simulink model "FOC_Ctrl_MBD"  (R2025b)
settings: Solver=FixedStepDiscrete  StartTime=0.0  StopTime=10.0  FixedStep=Ts  RelTol=1e-3
InitFcn:
  | mbd_s32k_consistency_checks(bdroot(gcs));
undefined symbols (not defined in the file): External, LQFP, One, Shot, TRGMUX_PDB_TRIG
libraries: mbd_s32k1xx_ec_toolbox x34, mbd_msd_ec_toolbox x1
settings Model: Creator=k  LastModifiedBy=k
settings SolverCC: AlgebraicLoopSolver=TrustRegion
settings DataIOCC: ExternalInput=off  InitialState=off  SaveOutput=off  SignalLogging=off  SaveTime=off
settings OptimizationCC: DefaultParameterBehavior=Inlined  StrengthReduction=on  PassReuseOutputArgsAs=Individual arguments  ZeroExternalMemoryAtStartup=off  ZeroInternalMemoryAtStartup=off  OptimizeBlockOrder=speed  OptimizationPriority=Speed  OptimizationCustomize=off  MultiThreadedLoops=on  AutoScheduleForLoops=on  EfficientTunableParamExpr=on
settings DebuggingCC: InheritedTsInSrcMsg=none  SingleTaskRateTransMsg=error  ParameterTunabilityLossMsg=error  UnconnectedInputMsg=error  UnconnectedOutputMsg=error  UnconnectedLineMsg=error  UnknownTsInhSupMsg=error
settings HardwareCC: ProdBitPerPointer=32.0  ProdBitPerSizeT=32.0  ProdBitPerPtrDiffT=32.0  ProdLargestAtomicInteger=Long  ProdLargestAtomicFloat=Double  ProdWordSize=32.0  ProdHWDeviceType=ARM Compatible->ARM Cortex
settings ModelReferenceCC: EnableRefExpFcnMdlSchedulingChecks=on  ModelReferenceNumInstancesAllowed=Single
settings SFSimCC: MATLABDynamicMemAlloc=off
settings RTWCC: SystemTargetFile=mbd_s32k.tlc  MakeCommand=mbd_s32k_make_rtw COPY_MDLREF_INCLUDES=0  TemplateMakefile=mbd_s32k.tmf  GenerateReport=on  GPUComputeCapability=3.5  DLArmComputeVersion=19.05  Description=Model Based Design Toolbox S32K1xx Code Generation Target
settings CodeAppCC: ForceParamTrailComments=on  IgnoreCustomStorageClasses=off  OperatorAnnotations=on  SimulinkDataObjDesc=on  SFDataObjDesc=on  InsertBlockDesc=on
settings STFCustomTargetCC: SystemTargetFile=mbd_s32k.tlc  TargetLangStandard=C99 (ISO)  MultiwordLength=256.0  ConcurrentExecutionCompliant=off  CombineOutputUpdateFcns=on  ERTCustomFileBanners=on  SubcomponentCodeInterfacePackaging=Nonreusable function  SupportContinuousTime=off  SupportNonInlinedSFcns=off  RemoveResetFunc=on  MATLABClassNameForMDSCustomization=Simulink.SoftwareTarget.ERTCustomization  GRTInterface=off
settings ERTTargetCC: ERTSrcFileBannerTemplate=mbd_ert_code_template.cgt  ERTHdrFileBannerTemplate=mbd_ert_code_template.cgt  ERTDataSrcFileTemplate=mbd_ert_code_template.cgt  ERTDataHdrFileTemplate=mbd_ert_code_template.cgt  ERTCustomFileTemplate=example_file_process.tlc  DynamicArrayContainerType=coder::array  TargetLangStandard=C99 (ISO)  ParMdlRefBuildCompliant=off  CompOptLevelCompliant=off  ConcurrentExecutionCompliant=off  SubcomponentCodeInterfacePackaging=Nonreusable function  ModelStepFunctionPrototypeControlCompliant=off  CPPClassGenCompliant=off  UseToolchainInfoCompliant=off

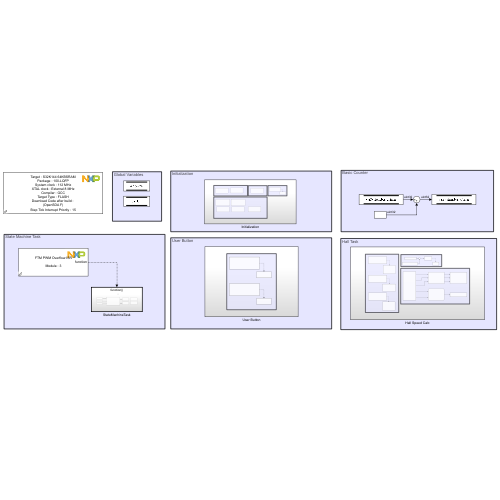
[thumbnail: Simulink's stored preview of the top-level diagram]
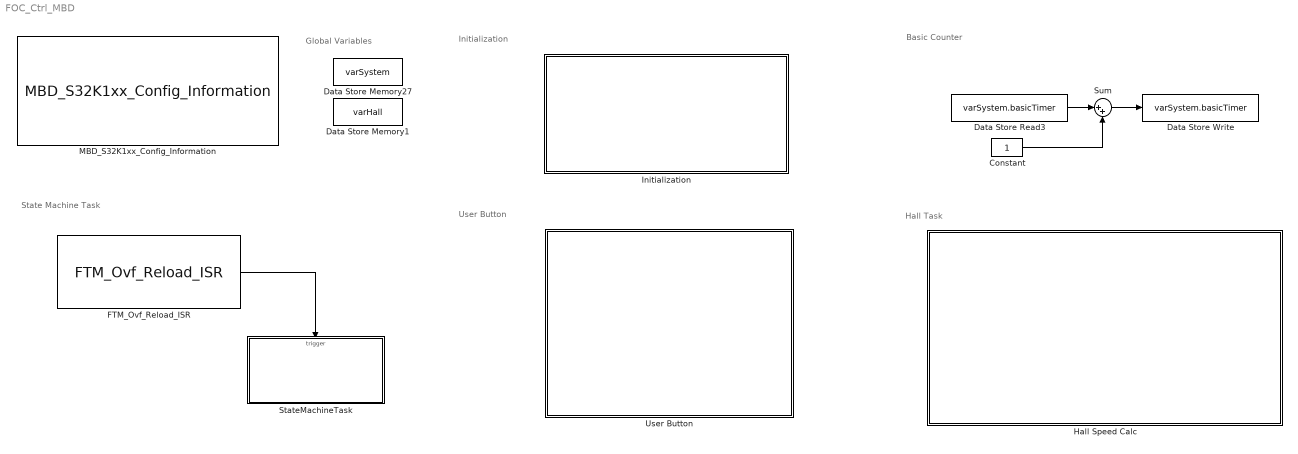
== system FOC_Ctrl_MBD ==
  note: Hall Task
  note: State Machine Task
  note: Global Variables
  note: User Button
  note: Initialization
  note: Basic Counter
  Constant : Constant  OutDataTypeStr=uint32
  Data Store Memory1 : DataStoreMemory  DataStoreName=varHall  ReadBeforeWriteMsg=warning  WriteAfterWriteMsg=warning  WriteAfterReadMsg=warning  ShowAdditionalParam=off  OutDataTypeStr=Bus: structHall
  Data Store Memory27 : DataStoreMemory  DataStoreName=varSystem  ReadBeforeWriteMsg=warning  WriteAfterWriteMsg=warning  WriteAfterReadMsg=warning  ShowAdditionalParam=off  OutDataTypeStr=Bus: structSystem
  Data Store Read3 : DataStoreRead  DataStoreName=varSystem  DataStoreElements=varSystem.basicTimer  IndexOptions=Index vector (dialog)  Indices=1  OutputSizes=1
  Data Store Write : DataStoreWrite  DataStoreName=varSystem  DataStoreElements=varSystem.basicTimer  IndexOptions=Index vector (dialog)  Indices=1  OutputSizes=1
  FTM_Ovf_Reload_ISR : mbd_s32k1xx_ec_toolbox/Motor Control Blocks/FTM Blocks/FTM_Ovf_Reload_ISR  Priority=10  ftmModule=3  mcuTargetUpdate=on
  Hall Speed Calc : Subsystem
  Initialization : Subsystem
  MBD_S32K1xx_Config_Information : mbd_s32k1xx_ec_toolbox/MBD_S32K1xx_Config_Information  mbdt_ver=0  disp_str=|  config_params=[]  mcu_target_name=S32K144  mcu_target_package=100-LQFP  mcu_target_sram_size=64KB  mcu_system_clock_freq=112  mcu_xtal_freq=External 8  mcu_steptick_timer=LPIT Channel 0  mcu_steptick_prio=15  ds_import_enable=on  target_compiler=GCC  target_memory=FLASH  gcc_target_compile_opts=-mthumb -mfloat-abi=hard -mfpu=fpv4-sp-d16 -O1 -g -gstrict-dwarf  gcc_target_assemble_opts=-mthumb -mfloat-abi=hard -mfpu=fpv4-sp-d16 -g  gcc_target_link_opts=-mthumb -mfloat-abi=hard -mfpu=fpv4-sp-d16  gcc_target_default_lcf=on  gcc_target_user_lcf=S32K144_64_flash.ld  ghs_target_compile_opts=-cpu=cortexm4f -thumb -fpu=vfpv4_d16 -fsingle -Ogeneral -Wundef -Wimplicit-int -Wshadow -Wtrigraphs --no_commons --gnu_asm -gnu99 -gdwarf-2 -G  ghs_target_assemble_opts=-cpu=cortexm4f -fpu=vfpv4_d16  ghs_target_link_opts=-cpu=cortexm4f -thumb -fpu=vfpv4_d16  ghs_target_default_lcf=on  ghs_target_user_lcf=S32K144_64_flash.ld  iar_target_compile_opts=--cpu=Cortex-M4F --thumb --fpu=VFPv4_sp -Ol -e --debug --dlib_config normal  iar_target_assemble_opts=--cpu Cortex-M4F --thumb --fpu VFPv4_sp  iar_target_link_opts=--no_exceptions --vfe --inline  iar_target_default_lcf=on  iar_target_user_lcf=S32K144_64_flash.icf  pil_download_enable=off  rbl_download_enable=on  rbl_start_delay=5000  rbl_download_interface=OpenSDA  rbl_restart_request=off  rbl_com_port=Custom  rbl_com_port_custom=COM1  pil_download_rate=57600  pil_download_rate_custom=115200  pil_opensda_drive=Custom  pil_opensda_drive_custom=F  jtag_interface=SEGGER JLink  jlink_default_path=off  jlink_user_path=C:\Program Files\SEGGER\JLink_V928  pil_uart_instance=1  pil_uart_rx=PTC6: [LPUART1_RX | Receive]  pil_uart_tx=PTC7: [LPUART1_TX | Transmit]  FTM_PWM_PcrCheckEnDis=on  FTM_Input_Edge_Inputs_PcrCheckEnDis=on  FTM_Dual_Edge_Inputs_PcrCheckEnDis=on  FTM_Quadrature_Inputs_PcrCheckEnDis=on  FTM_Hall_Sensor_Inputs_PcrCheckEnDis=on  LPTMR_PcrCheckEnDis=on  PIT_PcrCheckEnDis=on  RTC_PcrCheckEnDis=on  FlexCAN_PcrCheckEnDis=on  LIN_PcrCheckEnDis=on  FlexIO_PcrCheckEnDis=on  LPI2C_PcrCheckEnDis=on  LPSPI_PcrCheckEnDis=on  LPUART_PcrCheckEnDis=on  CMP_PcrCheckEnDis=on  GPIO_OutputPcrCheckEnDis=on  GPIO_InputPcrCheckEnDis=on  SBC_PcrCheckEnDis=on  BMS_PcrCheckEnDis=on  AMMCLIB_PcrCheckEnDis=on  FM_PcrCheckEnDis=on  Profile_PcrCheckEnDis=on  ConfigParams_PcrCheckEnDis=on  ModelRef_PcrCheckEnDis=on  PDB0_PcrCheckEnDis=on  CSEc_PcrCheckEnDis=on  eDMA_PcrCheckEnDis=on  FLASH_PcrCheckEnDis=on  ADC_PcrCheckEnDis=on  WDOG_PcrCheckEnDis=on
      | Target : S32K144-64KB_SRAM
      | Package : 100-pin
      | System clock : 80 MHz
      | XTAL clock : External 8 MHz
      | Compiler : IAR
      | Target Type : FLASH
      | Download Code after build : off
      | Step Tick Interrupt Priority : 15
  StateMachineTask : Subsystem
      settings: RTWSystemCode=Nonreusable function  RTWFileNameOpts=Use subsystem name  FunctionWithSeparateData=on
  Sum : Sum  Inputs=|++
  User Button : Subsystem
  wires:
  FTM_Ovf_Reload_ISR/1 -> StateMachineTask/Trigger
  Data Store Read3/1 -> Sum/1
  Constant/1 -> Sum/2
  Sum/1 -> Data Store Write/1

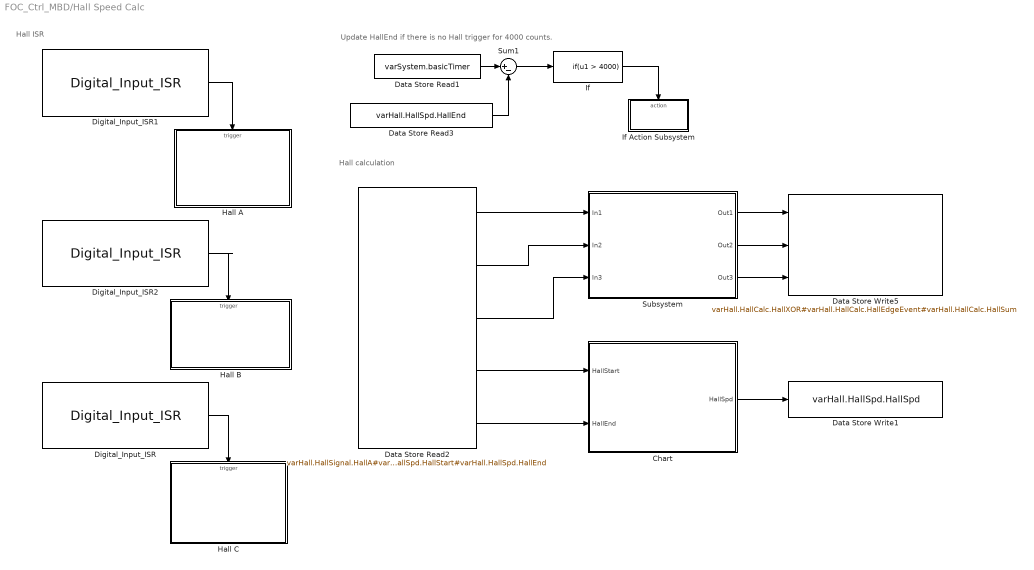
== system FOC_Ctrl_MBD/Hall Speed Calc ==
  note: Hall calculation
  note: Hall ISR
  note: Update HallEnd if there is no Hall trigger for 4000 counts.
  Chart : Stateflow chart  TreatAsAtomicUnit=on
  Data Store Read1 : DataStoreRead  DataStoreName=varSystem  DataStoreElements=varSystem.basicTimer  IndexOptions=Index vector (dialog)  Indices=1  OutputSizes=1
  Data Store Read2 : DataStoreRead  DataStoreName=varHall  DataStoreElements=varHall.HallSignal.HallA#varHall.HallSignal.HallB#varHall.HallSignal.HallC#varHall.HallSpd.HallStart#varHall.HallSpd.HallEnd  IndexOptions=Index vector (dialog)  Indices=1  OutputSizes=1
  Data Store Read3 : DataStoreRead  DataStoreName=varHall  DataStoreElements=varHall.HallSpd.HallEnd  IndexOptions=Index vector (dialog)  Indices=1  OutputSizes=1
  Data Store Write1 : DataStoreWrite  DataStoreName=varHall  DataStoreElements=varHall.HallSpd.HallSpd  IndexOptions=Index vector (dialog)  Indices=1  OutputSizes=1
  Data Store Write5 : DataStoreWrite  DataStoreName=varHall  DataStoreElements=varHall.HallCalc.HallXOR#varHall.HallCalc.HallEdgeEvent#varHall.HallCalc.HallSum  IndexOptions=Index vector (dialog)  Indices=1  OutputSizes=1
  Digital_Input_ISR : mbd_s32k1xx_ec_toolbox/GPIO Blocks/Digital_Input_ISR  gpio_pin=PTA1: [PTA1 | Port A I/O]  irqc=on either-edge  prio=5
  Digital_Input_ISR1 : mbd_s32k1xx_ec_toolbox/GPIO Blocks/Digital_Input_ISR  gpio_pin=PTA15: [PTA15 | Port A I/O]  irqc=on either-edge  prio=5
  Digital_Input_ISR2 : mbd_s32k1xx_ec_toolbox/GPIO Blocks/Digital_Input_ISR  gpio_pin=PTA16: [PTA16 | Port A I/O]  irqc=on either-edge  prio=5
  Hall A : Subsystem  TreatAsAtomicUnit=on
  Hall B : Subsystem  TreatAsAtomicUnit=on
  Hall C : Subsystem  TreatAsAtomicUnit=on
  If : If  IfExpression=u1 > 4000  ShowElse=off
  If Action Subsystem : Subsystem  TreatAsAtomicUnit=on
  Subsystem : Subsystem
  Sum1 : Sum  Inputs=|+-
  wires:
  Subsystem/1(Out1) -> Data Store Write5/1
  Subsystem/3(Out3) -> Data Store Write5/3
  Subsystem/2(Out2) -> Data Store Write5/2
  Chart/1(HallSpd) -> Data Store Write1/1
  Data Store Read2/3 -> Subsystem/3(In3)
  Data Store Read2/5 -> Chart/2(HallEnd)
  Data Store Read2/1 -> Subsystem/1(In1)
  Data Store Read2/2 -> Subsystem/2(In2)
  Data Store Read2/4 -> Chart/1(HallStart)
  Digital_Input_ISR2/1 -> Hall B/Trigger
  Digital_Input_ISR/1 -> Hall C/Trigger
  Digital_Input_ISR1/1 -> Hall A/Trigger
  Data Store Read1/1 -> Sum1/1
  Sum1/1 -> If/1
  Data Store Read3/1 -> Sum1/2
  If/1 -> If Action Subsystem/Action

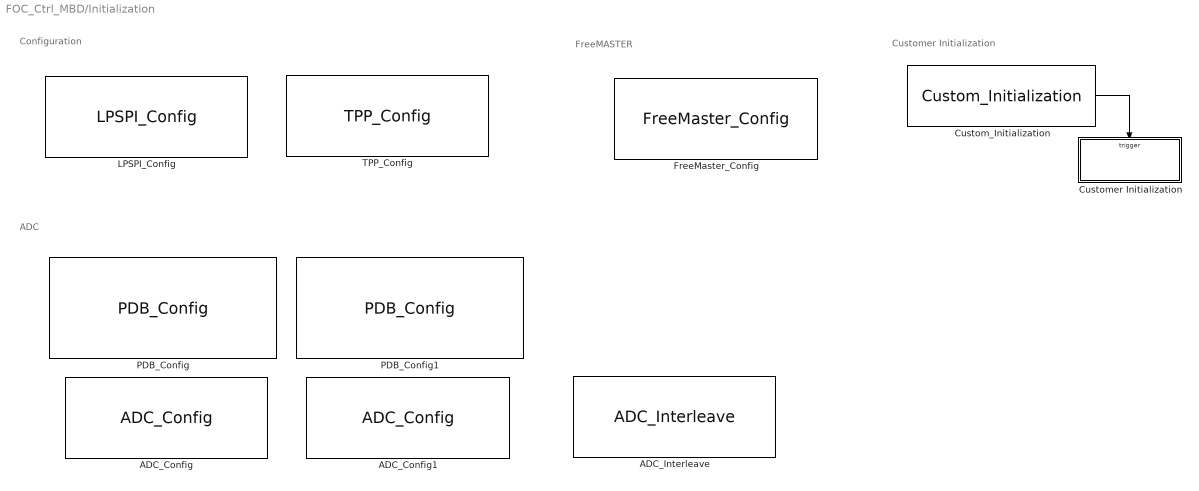
== system FOC_Ctrl_MBD/Initialization ==
  note: FreeMASTER
  note: ADC
  note: Configuration
  note: Customer Initialization
  ADC_Config : mbd_s32k1xx_ec_toolbox/Motor Control Blocks/ADC Blocks/ADC_Config  instance=0  mode=12-bit conversion  smplts=20  adiclk=alternate clock 1  adiv=input clock  show_adv_opts=on  pretrgsel=PDB pre-trigger  swpretrg=Disabled  adtrg=hardware  trgsel=PDB output  refsel=Vrefh and Vrefl  supply_monitoring=off  acfe=off  acfgt=off  acren=off  cv1=0  cv2=0  adco=off  avge=off  avgs=4 samples
  ADC_Config1 : mbd_s32k1xx_ec_toolbox/Motor Control Blocks/ADC Blocks/ADC_Config  instance=1  mode=12-bit conversion  smplts=20  adiclk=alternate clock 1  adiv=input clock  show_adv_opts=on  pretrgsel=PDB pre-trigger  swpretrg=Disabled  adtrg=hardware  trgsel=PDB output  refsel=Vrefh and Vrefl  supply_monitoring=off  acfe=off  acfgt=off  acren=off  cv1=0  cv2=0  adco=off  avge=off  avgs=4 samples
  ADC_Interleave : mbd_s32k1xx_ec_toolbox/Motor Control Blocks/ADC Blocks/ADC_Interleave  adcInterleavePins=PTB1 to ADC0_SE5 and ADC1_SE15  adcInterleaveInit=on
  Custom_Initialization : mbd_s32k1xx_ec_toolbox/Utility Blocks/Custom_Initialization
  Customer Initialization : Subsystem  TreatAsAtomicUnit=on
  FreeMaster_Config : mbd_s32k1xx_ec_toolbox/Utility Blocks/FreeMaster_Config  interface=LPUART1  baudrate=115200  rxd=PTC6: [LPUART1_RX | Receive]  txd=PTC7: [LPUART1_TX | Transmit]  mode=Poll-driven  isr_prio=15  show_adv_opts=on  use_scope=on  max_scope_vars=8  use_recorder=on  max_rec_vars=8  rec_buff_size=8192  rec_timebase=50 microseconds  comm_buffer_size_auto=on  comm_buffer_size=255  comm_rqueue_size_default=on  comm_rqueue_size=32
  "LPSPI_Config " : mbd_s32k1xx_ec_toolbox/Communication Blocks/SPI Blocks/LPSPI_Config   InstanceNumber=0  Role=Master  BaudRate=1000000  ShowAdvanced=on  sin=PTB3: [LPSPI0_SIN | LPSPI Serial Data Input]  sout=PTB4: [LPSPI0_SOUT | LPSPI Serial Data Output]  sck=PTB2: [LPSPI0_SCK | LPSPI Serial Clock I/O]  pcs0=None  pcs1=PTB5: [LPSPI0_PCS1 | Peripheral Chip Select 1]  pcs2=None  pcs3=None  CPHA=1  CPOL=0  BitOrder=MSB first  TransferSize=8  WhichPCS=0  PCSPol=ActiveLow  ContinuousTransfer=off
  PDB_Config : mbd_s32k1xx_ec_toolbox/Motor Control Blocks/PDB Blocks/PDB_Config  pdbModule=0  regScCont=One-Shot  regScTrgsel=External (TRGMUX_PDB_TRIG)  trgMuxSel=FTM3 Initialize Trigger  trgMuxSelPin=PTB5: [TRGMUX_IN0 | Trigger Mux Input]  regModModulus=6900  regScPrescaler=1  regScMult=1  regPoenPoen0=off  regPo0DlyDly1=0  regPo0DlyDly2=0  enable_pdb_init=on  show_adv_opts=on  regCh0C1En0=on  regCh0C1En1=on  regCh0C1En2=off  regCh0C1En3=off  regCh0C1En4=off  regCh0C1En5=off  regCh0C1En6=off  regCh0C1En7=off  regCh0C1Bb0=off  regCh0C1Bb1=off  regCh0C1Bb2=off  regCh0C1Bb3=off  regCh0C1Bb4=off  regCh0C1Bb5=off  regCh0C1Bb6=off  regCh0C1Bb7=off  regCh0C1Tos0=Pre-trigger is in delay mode  regCh0C1Tos1=Pre-trigger is in delay mode  regCh0C1Tos2=Pre-trigger is in delay mode  regCh0C1Tos3=Pre-trigger is in delay mode  regCh0C1Tos4=Pre-trigger is in delay mode  regCh0C1Tos5=Pre-trigger is in delay mode  regCh0C1Tos6=Pre-trigger is in delay mode  regCh0C1Tos7=Pre-trigger is in delay mode  regCh0DlyDly0=1750  regCh0DlyDly1=3500  regCh0DlyDly2=1000  regCh0DlyDly3=1500  regCh0DlyDly4=0  regCh0DlyDly5=0  regCh0DlyDly6=0  regCh0DlyDly7=0  regCh1C1En0=off  regCh1C1En1=off  regCh1C1En2=off  regCh1C1En3=off  regCh1C1En4=off  regCh1C1En5=off  regCh1C1En6=off  regCh1C1En7=off  regCh1C1Bb0=off  regCh1C1Bb1=off  regCh1C1Bb2=off  regCh1C1Bb3=off  regCh1C1Bb4=off  regCh1C1Bb5=off  regCh1C1Bb6=off  regCh1C1Bb7=off  regCh1C1Tos0=Pre-trigger is in delay mode  regCh1C1Tos1=Pre-trigger is in delay mode  regCh1C1Tos2=Pre-trigger is in delay mode  regCh1C1Tos3=Pre-trigger is in delay mode  regCh1C1Tos4=Pre-trigger is in delay mode  regCh1C1Tos5=Pre-trigger is in delay mode  regCh1C1Tos6=Pre-trigger is in delay mode  regCh1C1Tos7=Pre-trigger is in delay mode  regCh1DlyDly0=0  regCh1DlyDly1=0  regCh1DlyDly2=0  regCh1DlyDly3=0  regCh1DlyDly4=0  regCh1DlyDly5=0  regCh1DlyDly6=0  regCh1DlyDly7=0
  PDB_Config1 : mbd_s32k1xx_ec_toolbox/Motor Control Blocks/PDB Blocks/PDB_Config  pdbModule=1  regScCont=One-Shot  regScTrgsel=External (TRGMUX_PDB_TRIG)  trgMuxSel=FTM3 Initialize Trigger  trgMuxSelPin=PTB5: [TRGMUX_IN0 | Trigger Mux Input]  regModModulus=6900  regScPrescaler=1  regScMult=1  regPoenPoen0=off  regPo0DlyDly1=0  regPo0DlyDly2=0  enable_pdb_init=on  show_adv_opts=on  regCh0C1En0=on  regCh0C1En1=on  regCh0C1En2=on  regCh0C1En3=off  regCh0C1En4=off  regCh0C1En5=off  regCh0C1En6=off  regCh0C1En7=off  regCh0C1Bb0=off  regCh0C1Bb1=off  regCh0C1Bb2=off  regCh0C1Bb3=off  regCh0C1Bb4=off  regCh0C1Bb5=off  regCh0C1Bb6=off  regCh0C1Bb7=off  regCh0C1Tos0=Pre-trigger is in delay mode  regCh0C1Tos1=Pre-trigger is in delay mode  regCh0C1Tos2=Pre-trigger is in delay mode  regCh0C1Tos3=Pre-trigger is in delay mode  regCh0C1Tos4=Pre-trigger is in delay mode  regCh0C1Tos5=Pre-trigger is in delay mode  regCh0C1Tos6=Pre-trigger is in delay mode  regCh0C1Tos7=Pre-trigger is in delay mode  regCh0DlyDly0=1750  regCh0DlyDly1=2625  regCh0DlyDly2=3500  regCh0DlyDly3=0  regCh0DlyDly4=0  regCh0DlyDly5=0  regCh0DlyDly6=0  regCh0DlyDly7=0  regCh1C1En0=off  regCh1C1En1=off  regCh1C1En2=off  regCh1C1En3=off  regCh1C1En4=off  regCh1C1En5=off  regCh1C1En6=off  regCh1C1En7=off  regCh1C1Bb0=off  regCh1C1Bb1=off  regCh1C1Bb2=off  regCh1C1Bb3=off  regCh1C1Bb4=off  regCh1C1Bb5=off  regCh1C1Bb6=off  regCh1C1Bb7=off  regCh1C1Tos0=Pre-trigger is in delay mode  regCh1C1Tos1=Pre-trigger is in delay mode  regCh1C1Tos2=Pre-trigger is in delay mode  regCh1C1Tos3=Pre-trigger is in delay mode  regCh1C1Tos4=Pre-trigger is in delay mode  regCh1C1Tos5=Pre-trigger is in delay mode  regCh1C1Tos6=Pre-trigger is in delay mode  regCh1C1Tos7=Pre-trigger is in delay mode  regCh1DlyDly0=0  regCh1DlyDly1=0  regCh1DlyDly2=0  regCh1DlyDly3=0  regCh1DlyDly4=0  regCh1DlyDly5=0  regCh1DlyDly6=0  regCh1DlyDly7=0
  TPP_Config : mbd_msd_ec_toolbox/TPP/TPP_Config  Priority=1  tppInstance=0  desatMode=off  fullonMode=on  lockMode=on  overtempEvent=on  phaseEvent=on  desatEvent=on  framingEvent=on  vlsEvent=on  writeErrEvent=on  overcurrentEvent=on  resetEvent=on  mcuTppIntEn=off  prioInt=15  tppDeadtime=1000  initTppNow=on  tppSpiInst=0  tppPwmModule=3  tppPair0_1=on  tppPair2_3=on  tppPair4_5=on  tppPair6_7=off  tppFirstChHS=on  tppEn1Pin=PTA2: [PTA2 | Port A I/O]  tppEn2Pin=PTA2: [PTA2 | Port A I/O]  tppRstPin=PTA3: [PTA3 | Port A I/O]  tppCsPin=PTB5: [PTB5 | Port B I/O]  tppIntPin=PTE10: [PTE10 | Port E I/O]
  wires:
  Custom_Initialization/1 -> Customer Initialization/Trigger

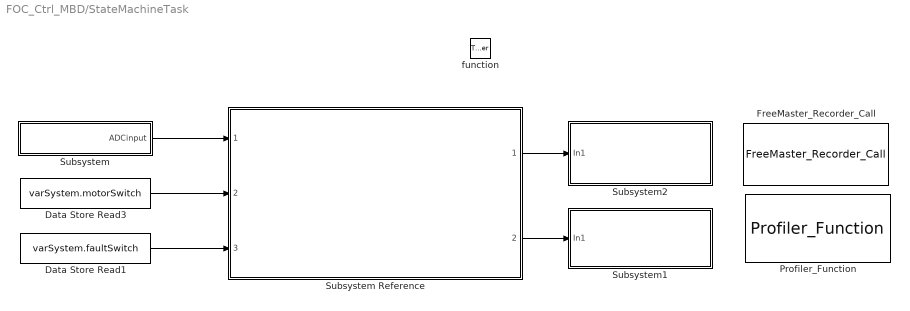
== system FOC_Ctrl_MBD/StateMachineTask ==
  function : TriggerPort  TriggerType=function-call  VariantControl=Variant
  Data Store Read1 : DataStoreRead  DataStoreName=varSystem  DataStoreElements=varSystem.faultSwitch  IndexOptions=Index vector (dialog)  Indices=1  OutputSizes=1
  Data Store Read3 : DataStoreRead  DataStoreName=varSystem  DataStoreElements=varSystem.motorSwitch  IndexOptions=Index vector (dialog)  Indices=1  OutputSizes=1
  FreeMaster_Recorder_Call : mbd_s32k1xx_ec_toolbox/Utility Blocks/FreeMaster_Recorder_Call
  Profiler_Function : mbd_s32k1xx_ec_toolbox/Utility Blocks/Profiler_Function  profile_indx=0
  Subsystem : Subsystem
  Subsystem Reference : Subsystem  ReferencedSubsystem=FOC_Sub_StateMch
  Subsystem1 : Subsystem
  Subsystem2 : Subsystem
  wires:
  Data Store Read3/1 -> Subsystem Reference/2
  Data Store Read1/1 -> Subsystem Reference/3
  Subsystem/1(ADCinput) -> Subsystem Reference/1
  Subsystem Reference/2 -> Subsystem1/1(In1)
  Subsystem Reference/1 -> Subsystem2/1(In1)

== system FOC_Ctrl_MBD/User Button ==
  note: User Button
  Button 1 : Subsystem  TreatAsAtomicUnit=on
  Button 2 : Subsystem  TreatAsAtomicUnit=on
  Digital_Input_ISR3 : mbd_s32k1xx_ec_toolbox/GPIO Blocks/Digital_Input_ISR  gpio_pin=PTC12: [PTC12 | Port C I/O]  irqc=on rising-edge  prio=13
  Digital_Input_ISR4 : mbd_s32k1xx_ec_toolbox/GPIO Blocks/Digital_Input_ISR  gpio_pin=PTC13: [PTC13 | Port C I/O]  irqc=on rising-edge  prio=13
  wires:
  Digital_Input_ISR3/1 -> Button 1/Trigger
  Digital_Input_ISR4/1 -> Button 2/Trigger

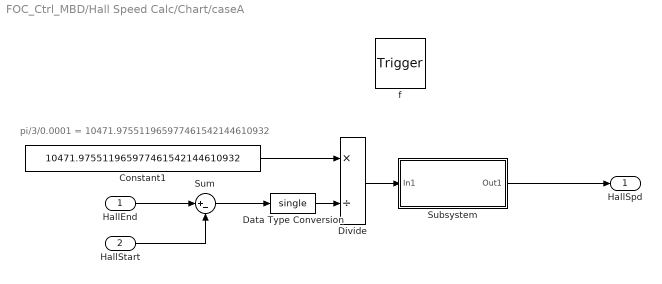
== system FOC_Ctrl_MBD/Hall Speed Calc/Chart/caseA ==
  note: pi/3/0.0001 = 10471.975511965977461542144610932
  HallEnd : Inport  OutDataTypeStr=uint32  PortDimensions=1
  HallStart : Inport  Port=2  OutDataTypeStr=uint32  PortDimensions=1
  f : TriggerPort  TriggerType=function-call  VariantControl=(inherit)
      settings: CopyFcn=Stateflow.SLINSF.SimulinkMan.removeBlockPreDeleteFcn  PreDeleteFcn=Stateflow.SLINSF.SimulinkMan.unsafePredeleteFcn
  Constant1 : Constant  Value=10471.975511965977461542144610932  OutDataTypeStr=single
  Data Type Conversion : DataTypeConversion  OutDataTypeStr=single  SaturateOnIntegerOverflow=off  RndMeth=Floor
  Divide : Product  Inputs=*/
  Subsystem : Subsystem
  Sum : Sum  Inputs=|+-
  HallSpd : Outport  OutDataTypeStr=single  PortDimensions=1
  wires:
  Constant1/1 -> Divide/1
  Subsystem/1(Out1) -> HallSpd/1
  Divide/1 -> Subsystem/1(In1)
  Sum/1 -> Data Type Conversion/1
  Data Type Conversion/1 -> Divide/2
  HallStart/1 -> Sum/2
  HallEnd/1 -> Sum/1

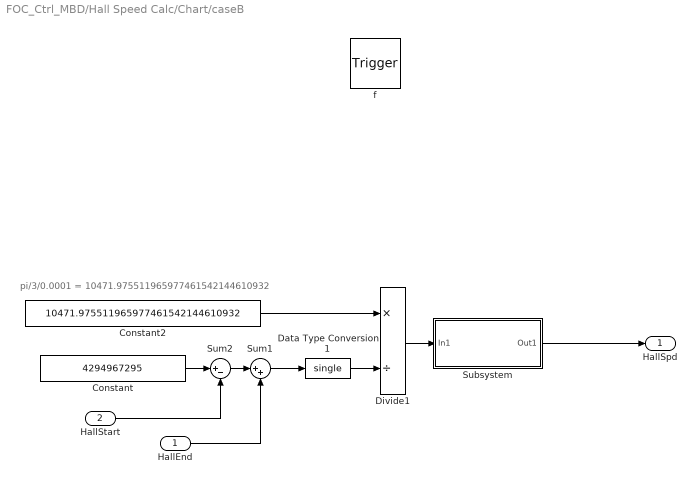
== system FOC_Ctrl_MBD/Hall Speed Calc/Chart/caseB ==
  note: pi/3/0.0001 = 10471.975511965977461542144610932
  HallEnd : Inport  OutDataTypeStr=uint32  PortDimensions=1
  HallStart : Inport  Port=2  OutDataTypeStr=uint32  PortDimensions=1
  f : TriggerPort  TriggerType=function-call  VariantControl=(inherit)
      settings: CopyFcn=Stateflow.SLINSF.SimulinkMan.removeBlockPreDeleteFcn  PreDeleteFcn=Stateflow.SLINSF.SimulinkMan.unsafePredeleteFcn
  Constant : Constant  Value=4294967295  OutDataTypeStr=uint32
  Constant2 : Constant  Value=10471.975511965977461542144610932  OutDataTypeStr=single
  Data Type Conversion1 : DataTypeConversion  OutDataTypeStr=single  SaturateOnIntegerOverflow=off  RndMeth=Floor
  Divide1 : Product  Inputs=*/
  Subsystem : Subsystem
  Sum1 : Sum  Inputs=|++
  Sum2 : Sum  Inputs=|+-
  HallSpd : Outport  OutDataTypeStr=single  PortDimensions=1
  wires:
  Subsystem/1(Out1) -> HallSpd/1
  Constant/1 -> Sum2/1
  Data Type Conversion1/1 -> Divide1/2
  Constant2/1 -> Divide1/1
  HallStart/1 -> Sum2/2
  Sum1/1 -> Data Type Conversion1/1
  Sum2/1 -> Sum1/1
  HallEnd/1 -> Sum1/2
  Divide1/1 -> Subsystem/1(In1)

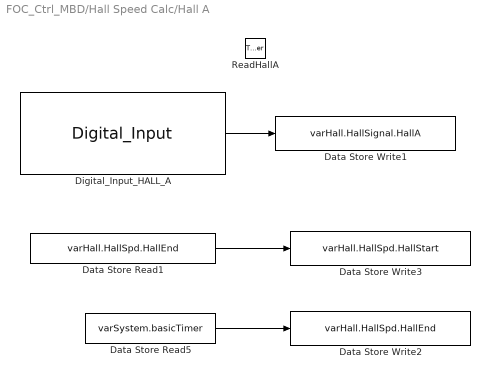
== system FOC_Ctrl_MBD/Hall Speed Calc/Hall A ==
  ReadHallA : TriggerPort  TriggerType=function-call  VariantControl=Variant
  Data Store Read1 : DataStoreRead  DataStoreName=varHall  DataStoreElements=varHall.HallSpd.HallEnd  IndexOptions=Index vector (dialog)  Indices=1  OutputSizes=1
  Data Store Read5 : DataStoreRead  DataStoreName=varSystem  DataStoreElements=varSystem.basicTimer  IndexOptions=Index vector (dialog)  Indices=1  OutputSizes=1
  Data Store Write1 : DataStoreWrite  DataStoreName=varHall  DataStoreElements=varHall.HallSignal.HallA  IndexOptions=Index vector (dialog)  Indices=1  OutputSizes=1
  Data Store Write2 : DataStoreWrite  DataStoreName=varHall  DataStoreElements=varHall.HallSpd.HallEnd  IndexOptions=Index vector (dialog)  Indices=1  OutputSizes=1
  Data Store Write3 : DataStoreWrite  DataStoreName=varHall  DataStoreElements=varHall.HallSpd.HallStart  IndexOptions=Index vector (dialog)  Indices=1  OutputSizes=1
  Digital_Input_HALL_A : mbd_s32k1xx_ec_toolbox/GPIO Blocks/Digital_Input  gpio_pin=PTA15: [PTA15 | Port A I/O]  pull_resistor=None  passive_filter=off
  wires:
  Digital_Input_HALL_A/1 -> Data Store Write1/1
  Data Store Read1/1 -> Data Store Write3/1
  Data Store Read5/1 -> Data Store Write2/1

== system FOC_Ctrl_MBD/Hall Speed Calc/Hall B ==
  ReadHallB : TriggerPort  TriggerType=function-call  VariantControl=Variant
  Data Store Read1 : DataStoreRead  DataStoreName=varHall  DataStoreElements=varHall.HallSpd.HallEnd  IndexOptions=Index vector (dialog)  Indices=1  OutputSizes=1
  Data Store Read5 : DataStoreRead  DataStoreName=varSystem  DataStoreElements=varSystem.basicTimer  IndexOptions=Index vector (dialog)  Indices=1  OutputSizes=1
  Data Store Write1 : DataStoreWrite  DataStoreName=varHall  DataStoreElements=varHall.HallSignal.HallB  IndexOptions=Index vector (dialog)  Indices=1  OutputSizes=1
  Data Store Write2 : DataStoreWrite  DataStoreName=varHall  DataStoreElements=varHall.HallSpd.HallEnd  IndexOptions=Index vector (dialog)  Indices=1  OutputSizes=1
  Data Store Write3 : DataStoreWrite  DataStoreName=varHall  DataStoreElements=varHall.HallSpd.HallStart  IndexOptions=Index vector (dialog)  Indices=1  OutputSizes=1
  Digital_Input_HALL_B : mbd_s32k1xx_ec_toolbox/GPIO Blocks/Digital_Input  gpio_pin=PTA16: [PTA16 | Port A I/O]  pull_resistor=None  passive_filter=off
  wires:
  Digital_Input_HALL_B/1 -> Data Store Write1/1
  Data Store Read5/1 -> Data Store Write2/1
  Data Store Read1/1 -> Data Store Write3/1

== system FOC_Ctrl_MBD/Hall Speed Calc/Hall C ==
  ReadHallC : TriggerPort  TriggerType=function-call  VariantControl=Variant
  Data Store Read1 : DataStoreRead  DataStoreName=varHall  DataStoreElements=varHall.HallSpd.HallEnd  IndexOptions=Index vector (dialog)  Indices=1  OutputSizes=1
  Data Store Read5 : DataStoreRead  DataStoreName=varSystem  DataStoreElements=varSystem.basicTimer  IndexOptions=Index vector (dialog)  Indices=1  OutputSizes=1
  Data Store Write1 : DataStoreWrite  DataStoreName=varHall  DataStoreElements=varHall.HallSignal.HallC  IndexOptions=Index vector (dialog)  Indices=1  OutputSizes=1
  Data Store Write2 : DataStoreWrite  DataStoreName=varHall  DataStoreElements=varHall.HallSpd.HallEnd  IndexOptions=Index vector (dialog)  Indices=1  OutputSizes=1
  Data Store Write3 : DataStoreWrite  DataStoreName=varHall  DataStoreElements=varHall.HallSpd.HallStart  IndexOptions=Index vector (dialog)  Indices=1  OutputSizes=1
  Digital_Input_HALL_C : mbd_s32k1xx_ec_toolbox/GPIO Blocks/Digital_Input  gpio_pin=PTA1: [PTA1 | Port A I/O]  pull_resistor=None  passive_filter=off
  wires:
  Digital_Input_HALL_C/1 -> Data Store Write1/1
  Data Store Read5/1 -> Data Store Write2/1
  Data Store Read1/1 -> Data Store Write3/1

== system FOC_Ctrl_MBD/Hall Speed Calc/If Action Subsystem ==
  Action Port : ActionPort  ActionPortLabel=if(u1 > 4000)
  Data Store Read5 : DataStoreRead  DataStoreName=varSystem  DataStoreElements=varSystem.basicTimer  IndexOptions=Index vector (dialog)  Indices=1  OutputSizes=1
  Data Store Write2 : DataStoreWrite  DataStoreName=varHall  DataStoreElements=varHall.HallSpd.HallEnd  IndexOptions=Index vector (dialog)  Indices=1  OutputSizes=1
  wires:
  Data Store Read5/1 -> Data Store Write2/1

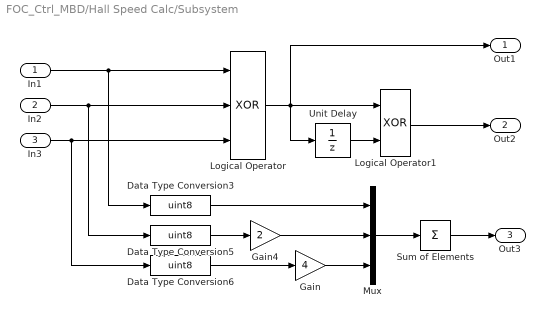
== system FOC_Ctrl_MBD/Hall Speed Calc/Subsystem ==
  In1 : Inport  PortDimensions=1
  In2 : Inport  Port=2  PortDimensions=1
  In3 : Inport  Port=3  PortDimensions=1
  Data Type Conversion3 : DataTypeConversion  OutDataTypeStr=uint8  SaturateOnIntegerOverflow=off  RndMeth=Floor
  Data Type Conversion5 : DataTypeConversion  OutDataTypeStr=uint8  SaturateOnIntegerOverflow=off  RndMeth=Floor
  Data Type Conversion6 : DataTypeConversion  OutDataTypeStr=uint8  SaturateOnIntegerOverflow=off  RndMeth=Floor
  Gain : Gain  Gain=4  OutDataTypeStr=uint8
  Gain4 : Gain  Gain=2  OutDataTypeStr=uint8
  Logical Operator : Logic  Operator=XOR  Inputs=3  AllPortsSameDT=off  OutDataTypeStr=boolean
  Logical Operator1 : Logic  Operator=XOR  AllPortsSameDT=off  OutDataTypeStr=boolean
  Mux : Mux  Inputs=3
  Sum of Elements : Sum  Inputs=+
  Unit Delay : UnitDelay  SampleTime=-1  HasFrameUpgradeWarning=on
  Out1 : Outport
  Out2 : Outport  Port=2
  Out3 : Outport  Port=3
  wires:
  Logical Operator1/1 -> Out2/1
  Sum of Elements/1 -> Out3/1
  In2/1 -> Logical Operator/2, Data Type Conversion5/1
  Data Type Conversion5/1 -> Gain4/1
  Mux/1 -> Sum of Elements/1
  In1/1 -> Logical Operator/1, Data Type Conversion3/1
  Gain/1 -> Mux/3
  Data Type Conversion3/1 -> Mux/1
  Data Type Conversion6/1 -> Gain/1
  In3/1 -> Logical Operator/3, Data Type Conversion6/1
  Logical Operator/1 -> Logical Operator1/1, Unit Delay/1, Out1/1
  Unit Delay/1 -> Logical Operator1/2
  Gain4/1 -> Mux/2

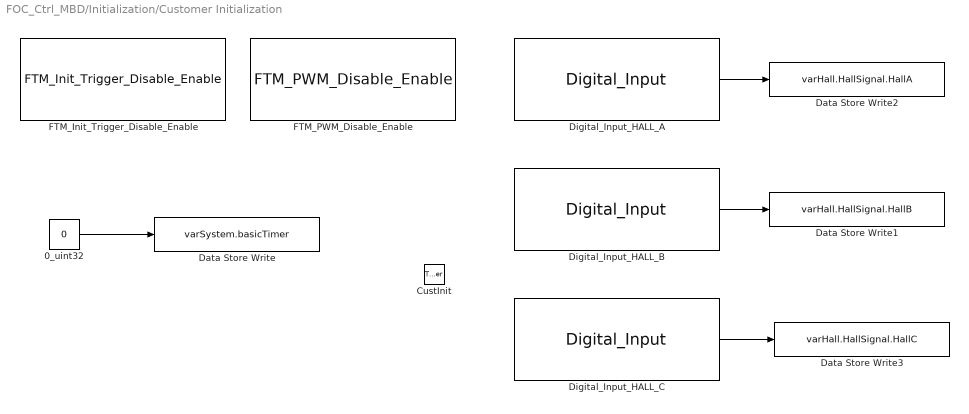
== system FOC_Ctrl_MBD/Initialization/Customer Initialization ==
  CustInit : TriggerPort  TriggerType=function-call  VariantControl=Variant
  0_uint32 : Constant  Value=0  OutDataTypeStr=uint32
  Data Store Write : DataStoreWrite  DataStoreName=varSystem  DataStoreElements=varSystem.basicTimer  IndexOptions=Index vector (dialog)  Indices=1  OutputSizes=1
  Data Store Write1 : DataStoreWrite  DataStoreName=varHall  DataStoreElements=varHall.HallSignal.HallB  IndexOptions=Index vector (dialog)  Indices=1  OutputSizes=1
  Data Store Write2 : DataStoreWrite  DataStoreName=varHall  DataStoreElements=varHall.HallSignal.HallA  IndexOptions=Index vector (dialog)  Indices=1  OutputSizes=1
  Data Store Write3 : DataStoreWrite  DataStoreName=varHall  DataStoreElements=varHall.HallSignal.HallC  IndexOptions=Index vector (dialog)  Indices=1  OutputSizes=1
  Digital_Input_HALL_A : mbd_s32k1xx_ec_toolbox/GPIO Blocks/Digital_Input  gpio_pin=PTA15: [PTA15 | Port A I/O]  pull_resistor=None  passive_filter=off
  Digital_Input_HALL_B : mbd_s32k1xx_ec_toolbox/GPIO Blocks/Digital_Input  gpio_pin=PTA16: [PTA16 | Port A I/O]  pull_resistor=None  passive_filter=off
  Digital_Input_HALL_C : mbd_s32k1xx_ec_toolbox/GPIO Blocks/Digital_Input  gpio_pin=PTA1: [PTA1 | Port A I/O]  pull_resistor=None  passive_filter=off
  FTM_Init_Trigger_Disable_Enable : mbd_s32k1xx_ec_toolbox/Motor Control Blocks/FTM Blocks/FTM_Init_Trigger_Disable_Enable  ftmModule=3  action=Enable
  FTM_PWM_Disable_Enable : mbd_s32k1xx_ec_toolbox/Motor Control Blocks/FTM Blocks/FTM_PWM_Disable_Enable  ftmModule=3  action=Enable
  wires:
  Digital_Input_HALL_A/1 -> Data Store Write2/1
  Digital_Input_HALL_C/1 -> Data Store Write3/1
  Digital_Input_HALL_B/1 -> Data Store Write1/1
  0_uint32/1 -> Data Store Write/1

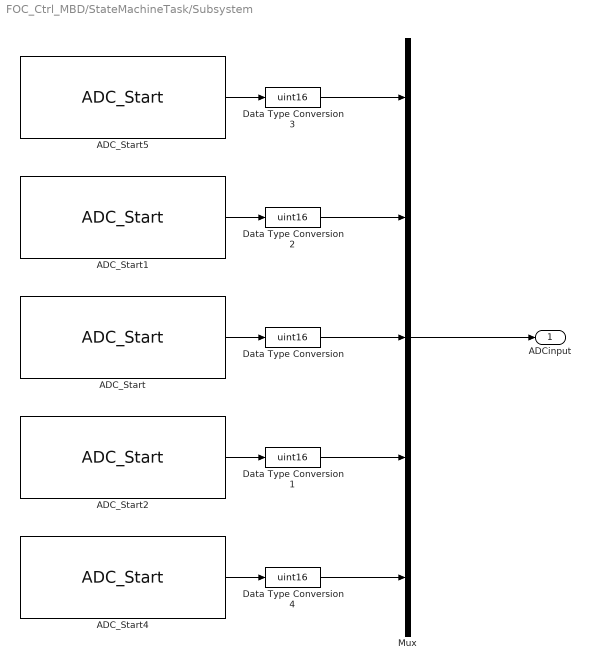
== system FOC_Ctrl_MBD/StateMachineTask/Subsystem ==
  ADC_Start : mbd_s32k1xx_ec_toolbox/Motor Control Blocks/ADC Blocks/ADC_Start  instance=1  adc_r=A  adc_chan=PTD4: [ADC1_SE6 | ADC Single Ended Input]  aien=off  mcuTargetUpdate=on
  ADC_Start1 : mbd_s32k1xx_ec_toolbox/Motor Control Blocks/ADC Blocks/ADC_Start  instance=1  adc_r=C  adc_chan=PTB1: [ADC1_SE15 | ADC Single Ended Input]  aien=off  mcuTargetUpdate=on
  ADC_Start2 : mbd_s32k1xx_ec_toolbox/Motor Control Blocks/ADC Blocks/ADC_Start  instance=1  adc_r=B  adc_chan=PTB12: [ADC1_SE7 | ADC Single Ended Input]  aien=off  mcuTargetUpdate=on
  ADC_Start4 : mbd_s32k1xx_ec_toolbox/Motor Control Blocks/ADC Blocks/ADC_Start  instance=0  adc_r=A  adc_chan=PTC14: [ADC0_SE12 | ADC Single Ended Input]  aien=off  mcuTargetUpdate=on
  ADC_Start5 : mbd_s32k1xx_ec_toolbox/Motor Control Blocks/ADC Blocks/ADC_Start  instance=0  adc_r=B  adc_chan=PTB0: [ADC0_SE4 | ADC Single Ended Input]  aien=off  mcuTargetUpdate=on
  Data Type Conversion{,1..4} (5 alike) : DataTypeConversion  OutDataTypeStr=uint16  SaturateOnIntegerOverflow=off  RndMeth=Floor
  Mux : Mux  Inputs=5
  ADCinput : Outport  OutDataTypeStr=uint16  PortDimensions=5
  wires:
  Data Type Conversion3/1 -> Mux/1
  ADC_Start1/1 -> Data Type Conversion2/1
  ADC_Start/1 -> Data Type Conversion/1
  Data Type Conversion4/1 -> Mux/5
  Data Type Conversion/1 -> Mux/3
  ADC_Start4/1 -> Data Type Conversion4/1
  ADC_Start5/1 -> Data Type Conversion3/1
  Data Type Conversion2/1 -> Mux/2
  ADC_Start2/1 -> Data Type Conversion1/1
  Data Type Conversion1/1 -> Mux/4
  Mux/1 -> ADCinput/1

== system FOC_Ctrl_MBD/StateMachineTask/Subsystem1 ==
  In1 : Inport  PortDimensions=3
  Demux : Demux  Outputs=3
  LED_Blue : mbd_s32k1xx_ec_toolbox/GPIO Blocks/Digital_Output  gpio_pin=PTD0: [PTD0 | Port D I/O]  init_val=High  drive_strength=Low
  LED_Green : mbd_s32k1xx_ec_toolbox/GPIO Blocks/Digital_Output  gpio_pin=PTD16: [PTD16 | Port D I/O]  init_val=High  drive_strength=Low
  LED_Red : mbd_s32k1xx_ec_toolbox/GPIO Blocks/Digital_Output  gpio_pin=PTD15: [PTD15 | Port D I/O]  init_val=High  drive_strength=Low
  wires:
  Demux/3 -> LED_Blue/1
  Demux/1 -> LED_Red/1
  Demux/2 -> LED_Green/1
  In1/1 -> Demux/1

== system FOC_Ctrl_MBD/StateMachineTask/Subsystem2 ==
  In1 : Inport  PortDimensions=3
  Demux : Demux  Outputs=3
  FTM_PWM_Config1 : mbd_s32k1xx_ec_toolbox/Motor Control Blocks/FTM Blocks/FTM_PWM_Config  Priority=5  ftmModule=3  ftmMode=Center-Aligned PWM  ftmSourceClock=112 MHz  swcontrol_enable=off  chan0En=on  chan0Type=Complementary  chan2En=on  chan2Type=Complementary  chan4En=on  chan4Type=Complementary  chan6En=off  chan6Type=Independent  ftmPwmUnits=Hz  outFrequency=16000  ftmPeriod=7000  ftmPrescaler=Divide by 1  deadtimeUnits=Nanoseconds  deadtimeNs=1000  deadtimeTicks=28  deadtimePrescaler=Divide by 4  dutyCycleCh0=0  dutyCycleCh1=0  dutyCycleCh2=0  dutyCycleCh3=0  dutyCycleCh4=0  dutyCycleCh5=0  dutyCycleCh6=0.25  dutyCycleCh7=0.25  dutyCycleSim=off  startAfterInit=off  showAdvOpt=on  pinFtmCh0=PTB8: [FTM3_CH0 | FTM Channel]  pinFtmCh1=PTB9: [FTM3_CH1 | FTM Channel]  pinPolCh0=Active Low  pinPolCh1=Active Low  outputComplem0=Main duplicated  outputLevel0=High  outputLevel1=Low  pinFtmCh2=PTB10: [FTM3_CH2 | FTM Channel]  pinFtmCh3=PTB11: [FTM3_CH3 | FTM Channel]  pinPolCh2=Active Low  pinPolCh3=Active Low  outputComplem2=Main duplicated  outputLevel2=High  outputLevel3=Low  pinFtmCh4=PTC10: [FTM3_CH4 | FTM Channel]  pinFtmCh5=PTC11: [FTM3_CH5 | FTM Channel]  pinPolCh4=Active Low  pinPolCh5=Active Low  outputComplem4=Main duplicated  outputLevel4=High  outputLevel5=Low  pinFtmCh6=PTC12: [FTM3_CH6 | FTM Channel]  pinFtmCh7=None  pinPolCh6=Active Low  pinPolCh7=Active Low  outputComplem6=Main duplicated  outputLevel6=Low  outputLevel7=Low  initTrigger=off  chTrigger0=off  chTrigger1=off  chTrigger2=off  chTrigger3=off  chTrigger4=off  chTrigger5=off  chTrigger6=off  chTrigger7=off  mcuTargetUpdate=on  pwmSyncTrg=Software trigger  pwmSyncHwRouting=TRGMUX_FTM7  pwmSyncTrg0=off  pwmSyncTrg1=off  pwmSyncTrg2=off  pwmSyncAutoClear=off  pwmSyncMinLoad=on  pwmSyncMaxLoad=off  pwmSyncInvert=PWM Syncronization  pwmSyncOutControl=System Clock  pwmSyncOutMask=System Clock  pwmSyncCounterInitial=PWM Syncronization  pwmSyncPoints=Wait Loading Points  reloadEnable=on  reloadPriority=5  reloadHalfCycle=off  reloadHCR=0  reloadFrequency=0  chnMatch0=off  chnMatch1=off  chnMatch2=off  chnMatch3=off  chnMatch4=off  chnMatch5=off  chnMatch6=off  chnMatch7=off  pwmFaultProtection=off  pwmFaultInterrupt=off  pwmFaultClearing=Fault control disabled  pwmFaultPinState=Safe Value  pwmFaultFilterValue=0  pwmFaultPriority=15  fault_disen_0=off  fault_filter_0=off  fault_polarity_0=Active High  fault_disen_1=off  fault_filter_1=off  fault_polarity_1=Active high  fault_disen_2=off  fault_filter_2=off  fault_polarity_2=Active high  fault_disen_3=off  fault_filter_3=off  fault_polarity_3=Active high  fault_pin_0=None  fault_pin_1=None  fault_pin_2=None  fault_pin_3=None
  wires:
  Demux/3 -> FTM_PWM_Config1/3
  In1/1 -> Demux/1
  Demux/1 -> FTM_PWM_Config1/1
  Demux/2 -> FTM_PWM_Config1/2

== system FOC_Ctrl_MBD/User Button/Button 1 ==
  Button1 : TriggerPort  TriggerType=function-call  VariantControl=Variant
  Data Store Read : DataStoreRead  DataStoreName=varSystem  DataStoreElements=varSystem.motorSwitch  IndexOptions=Index vector (dialog)  Indices=1  OutputSizes=1
  Data Store Write : DataStoreWrite  DataStoreName=varSystem  DataStoreElements=varSystem.motorSwitch  IndexOptions=Index vector (dialog)  Indices=1  OutputSizes=1
  Logical Operator : Logic  Operator=NOT  AllPortsSameDT=off  OutDataTypeStr=boolean
  wires:
  Logical Operator/1 -> Data Store Write/1
  Data Store Read/1 -> Logical Operator/1

== system FOC_Ctrl_MBD/User Button/Button 2 ==
  Button2 : TriggerPort  TriggerType=function-call  VariantControl=Variant
  Data Store Read : DataStoreRead  DataStoreName=varSystem  DataStoreElements=varSystem.faultSwitch  IndexOptions=Index vector (dialog)  Indices=1  OutputSizes=1
  Data Store Write : DataStoreWrite  DataStoreName=varSystem  DataStoreElements=varSystem.faultSwitch  IndexOptions=Index vector (dialog)  Indices=1  OutputSizes=1
  Logical Operator : Logic  Operator=NOT  AllPortsSameDT=off  OutDataTypeStr=boolean
  wires:
  Data Store Read/1 -> Logical Operator/1
  Logical Operator/1 -> Data Store Write/1

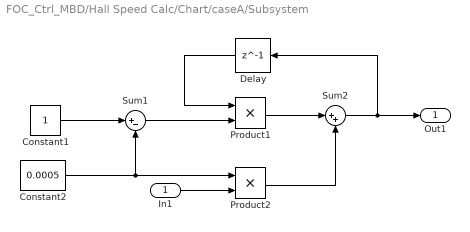
== system FOC_Ctrl_MBD/Hall Speed Calc/Chart/caseA/Subsystem ==
  In1 : Inport
  Constant1 : Constant  OutDataTypeStr=single
  Constant2 : Constant  Value=0.0005  OutDataTypeStr=single
  Delay : Delay  DelayLength=1  InitialCondition=0
  Product1 : Product
  Product2 : Product
  Sum1 : Sum  Inputs=|+-
  Sum2 : Sum  Inputs=|++
  Out1 : Outport
  wires:
  In1/1 -> Product2/2
  Product2/1 -> Sum2/2
  Sum2/1 -> Delay/1, Out1/1
  Product1/1 -> Sum2/1
  Constant1/1 -> Sum1/1
  Constant2/1 -> Product2/1, Sum1/2
  Sum1/1 -> Product1/2
  Delay/1 -> Product1/1

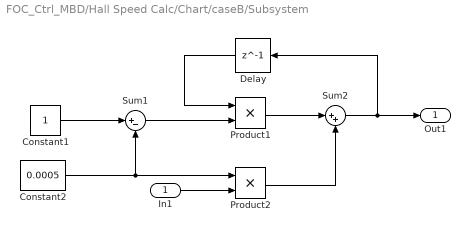
== system FOC_Ctrl_MBD/Hall Speed Calc/Chart/caseB/Subsystem ==
  In1 : Inport
  Constant1 : Constant  OutDataTypeStr=single
  Constant2 : Constant  Value=0.0005  OutDataTypeStr=single
  Delay : Delay  DelayLength=1  InitialCondition=0
  Product1 : Product
  Product2 : Product
  Sum1 : Sum  Inputs=|+-
  Sum2 : Sum  Inputs=|++
  Out1 : Outport
  wires:
  In1/1 -> Product2/2
  Product2/1 -> Sum2/2
  Sum2/1 -> Delay/1, Out1/1
  Product1/1 -> Sum2/1
  Constant1/1 -> Sum1/1
  Constant2/1 -> Product2/1, Sum1/2
  Sum1/1 -> Product1/2
  Delay/1 -> Product1/1

== stateflow chart FOC_Ctrl_MBD/Hall Speed Calc/Chart ==
  state HallSpd = caseA(HallEnd,HallStart) [function]
  state HallSpd = caseB(HallEnd,HallStart) [function]
  (default) -> (junction 3)
  (junction 3) -> (junction 5) [order 1] : [HallStart < HallEnd]
  (junction 5) -> (junction 14) : {HallSpd = caseA(HallEnd, HallStart);}
  (junction 3) -> (junction 7) [order 2]
  (junction 7) -> (junction 9) [order 1] : [HallStart == HallEnd]
  (junction 9) -> (junction 19) : {HallSpd = 0;}
  (junction 7) -> (junction 11) [order 2]
  (junction 11) -> (junction 21) : {HallSpd = caseB(HallEnd, HallStart);}
  data: HallEnd function_input uint32 size=1; HallStart function_input uint32 size=1; HallSpd function_output single size=1; HallEnd function_input uint32 size=1; HallStart function_input uint32 size=1; HallSpd function_output single size=1; HallStart input uint32 size=1; HallEnd input uint32 size=1; HallSpd output single size=1
